simulink model "PID_controller_open_loop"  (R2016a)
settings: Solver=VariableStepAuto  StartTime=0.0  StopTime=10.0  RelTol=1e-3
values from neighbouring files (symbols this model uses):
  Ki_theta = par_pid(i,2)    [PID_robstab.m]    (also in PID_wcp.m; err_fun.m = par(:,2); sim_MC_PID.m = par_pid(3,2); sim_PID_pendulum_nominal.m = par_pid(3,2))
  Kp = par_pid(i,4)    [PID_robstab.m]    (also in PID_wcp.m; err_fun.m = par(:,4); sim_MC_PID.m = par_pid(3,4); sim_PID_pendulum_nominal.m = par_pid(3,4))
  Kp_theta = par_pid(i,1)    [PID_robstab.m]    (also in PID_wcp.m; err_fun.m = par(:,1); sim_MC_PID.m = par_pid(3,1); sim_PID_pendulum_nominal.m = par_pid(3,1))
  N = par_pid(i,7)    [PID_robstab.m]    (also in PID_wcp.m; err_fun.m = par(:,7); sim_MC_PID.m = par_pid(3,7); sim_PID_pendulum_nominal.m = par_pid(3,7))
  N_theta = par_pid(i,6)    [PID_robstab.m]    (also in PID_wcp.m; err_fun.m = par(:,6); sim_MC_PID.m = par_pid(3,6); sim_PID_pendulum_nominal.m = par_pid(3,6))
  Td = par_pid(i,5)    [PID_robstab.m]    (also in PID_wcp.m; err_fun.m = par(:,5); sim_MC_PID.m = par_pid(3,5); sim_PID_pendulum_nominal.m = par_pid(3,5))
  Td_theta = par_pid(i,3)    [PID_robstab.m]    (also in PID_wcp.m; err_fun.m = par(:,3); sim_MC_PID.m = par_pid(3,3); sim_PID_pendulum_nominal.m = par_pid(3,3))
undefined symbols (not defined in the file or in its folder): DiscIntNeverNeededParam
settings Model: Creator=ts_slavov  LastModifiedBy=ts_slavov

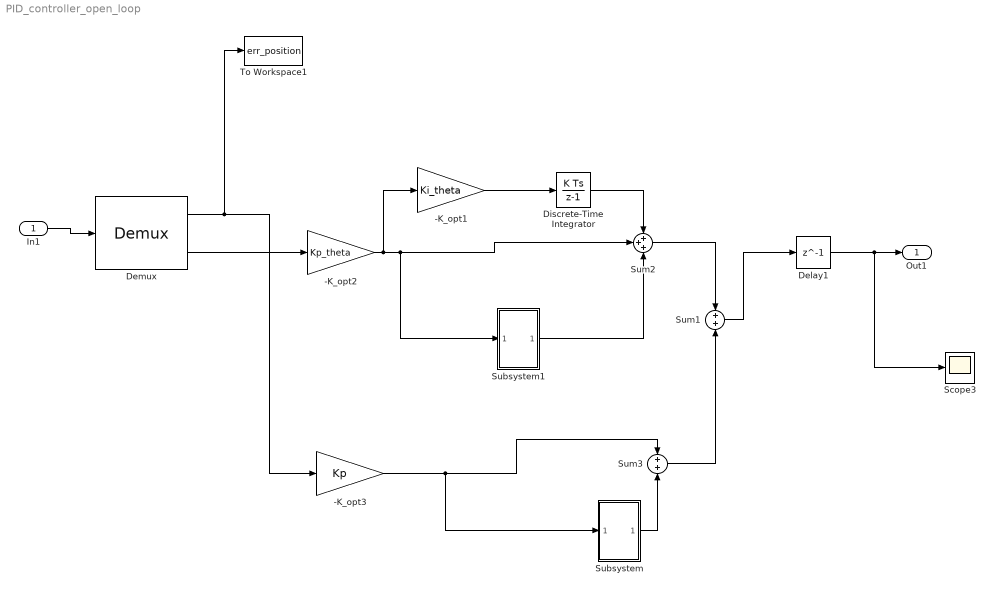
== system PID_controller_open_loop ==
  In1 : Inport  OutDataTypeStr=double
  -K_opt1 : Gain  Gain=Ki_theta  OutDataTypeStr=double  RndMeth=Round  SaturateOnIntegerOverflow=on
  -K_opt2 : Gain  Gain=Kp_theta  OutDataTypeStr=double  RndMeth=Round  SaturateOnIntegerOverflow=on
  -K_opt3 : Gain  Gain=Kp  OutDataTypeStr=double  RndMeth=Round  SaturateOnIntegerOverflow=on
  Delay1 : Delay  DelayLength=1  SampleTime=0.01
  Demux : Demux  Outputs=2
  Discrete-Time Integrator : DiscreteIntegrator  InitialConditionSetting=State (most efficient)  SampleTime=0.01  ICPrevOutput=DiscIntNeverNeededParam  ICPrevScaledInput=DiscIntNeverNeededParam
  Scope3 : Scope
  Subsystem : Subsystem
  Subsystem1 : Subsystem
  Sum1 : Sum
  Sum2 : Sum  Inputs=+++
  Sum3 : Sum
  To Workspace1 : ToWorkspace  VariableName=err_position  SampleTime=-1
      settings: Save2DSignal=2-D array (concatenate along first dimension)
  Out1 : Outport  OutDataTypeStr=double
  wires:
  Demux/1 -> To Workspace1/1, -K_opt3/1
  In1/1 -> Demux/1
  Sum2/1 -> Sum1/1
  Demux/2 -> -K_opt2/1
  Discrete-Time Integrator/1 -> Sum2/1
  Subsystem1/1(Out1) -> Sum2/3
  -K_opt2/1 -> -K_opt1/1, Subsystem1/1(In1), Sum2/2
  -K_opt1/1 -> Discrete-Time Integrator/1
  -K_opt3/1 -> Subsystem/1(In1), Sum3/1
  Subsystem/1(Out1) -> Sum3/2
  Sum3/1 -> Sum1/2
  Sum1/1 -> Delay1/1
  Delay1/1 -> Scope3/1, Out1/1

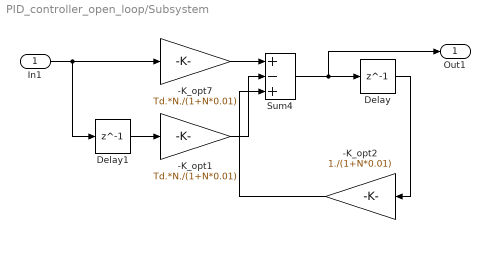
== system PID_controller_open_loop/Subsystem ==
  In1 : Inport  OutDataTypeStr=double
  -K_opt1 : Gain  Gain=Td.*N./(1+N*0.01)  OutDataTypeStr=double  RndMeth=Round  SaturateOnIntegerOverflow=on
  -K_opt2 : Gain  Gain=1./(1+N*0.01)  OutDataTypeStr=double  RndMeth=Round  SaturateOnIntegerOverflow=on
  -K_opt7 : Gain  Gain=Td.*N./(1+N*0.01)  OutDataTypeStr=double  RndMeth=Round  SaturateOnIntegerOverflow=on
  Delay : Delay  DelayLength=1  SampleTime=0.01
  Delay1 : Delay  DelayLength=1  SampleTime=0.01
  Sum4 : Sum  Inputs=+-+
  Out1 : Outport  OutDataTypeStr=double
  wires:
  -K_opt2/1 -> Sum4/3
  Delay/1 -> -K_opt2/1
  -K_opt1/1 -> Sum4/2
  Sum4/1 -> Delay/1, Out1/1
  Delay1/1 -> -K_opt1/1
  -K_opt7/1 -> Sum4/1
  In1/1 -> -K_opt7/1, Delay1/1

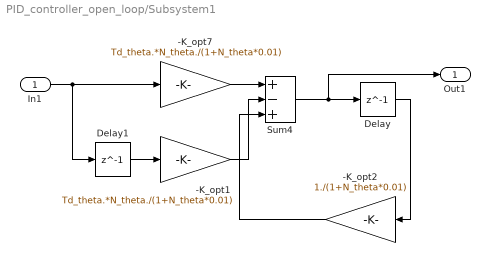
== system PID_controller_open_loop/Subsystem1 ==
  In1 : Inport  OutDataTypeStr=double
  -K_opt1 : Gain  Gain=Td_theta.*N_theta./(1+N_theta*0.01)  OutDataTypeStr=double  RndMeth=Round  SaturateOnIntegerOverflow=on
  -K_opt2 : Gain  Gain=1./(1+N_theta*0.01)  OutDataTypeStr=double  RndMeth=Round  SaturateOnIntegerOverflow=on
  -K_opt7 : Gain  Gain=Td_theta.*N_theta./(1+N_theta*0.01)  OutDataTypeStr=double  RndMeth=Round  SaturateOnIntegerOverflow=on
  Delay : Delay  DelayLength=1  SampleTime=0.01
  Delay1 : Delay  DelayLength=1  SampleTime=0.01
  Sum4 : Sum  Inputs=+-+
  Out1 : Outport  OutDataTypeStr=double
  wires:
  In1/1 -> Delay1/1, -K_opt7/1
  -K_opt7/1 -> Sum4/1
  Delay1/1 -> -K_opt1/1
  Sum4/1 -> Out1/1, Delay/1
  -K_opt1/1 -> Sum4/2
  Delay/1 -> -K_opt2/1
  -K_opt2/1 -> Sum4/3
